simulink model "Mass_Springs_Systems"  (R2021b)
settings: Solver=ode4  StartTime=0.0  StopTime=20  FixedStep=.001  RelTol=1e-3  AbsTol=1e-3  EnableMultiTasking=on
model workspace (MAT data in the model file):
  cslide = 0.25
  iz = [0.192  0.091; 0.207  0.094; 0.221  0.104; 0.238  0.118; 0.251  0.141; 0.262  0.168; 0.268  0.205; 0.27  0.242; 0.267  0.277; 0.262  0.308; 0.246  0.348; 0.232  0.369; 0.206  0.39; 0.185  0.39; 0.16  0.377; 0.137  0.349; 0.126  0.325; 0.118  0.297; 0.114  0.265; 0.113  0.237; 0.118  0.191; 0.128  0.156; 0.139  0.13; 0.156  0.107; 0.175  0.096]
  m1 = 0
  m2 = 0
  m3 = 0
  one = [0.064  0.072; 0.088  0.03; 0.169  0.03; 0.168  0.458; 0.129  0.458; 0.128  0.073]
  smiData.RigidTransform.translation = [-21.5561986301 -14.8674859839 15.0728144895]
  smiData.RigidTransform.angle = 0
  smiData.RigidTransform.axis = [0 0 0]
  smiData.RigidTransform.ID = 'RootGround[rack-1]'
  smiData.Solid.mass = 0.0200061588425
  smiData.Solid.CoM = [0 0.838779102261 -0.00603396973069]
  smiData.Solid.MoI = [0.670200057653 0.669872690066 0.00366172739385]
  smiData.Solid.PoI = [5.56695055283e-05 0 0]
  smiData.Solid.color = [0.792156862745 0.819607843137 0.933333333333]
  smiData.Solid.opacity = 1
  smiData.Solid.ID = 'rack*:*Default'
  three = [0.252  0.12; 0.239  0.091; 0.214  0.068; 0.179  0.053; 0.14  0.052; 0.107  0.064; 0.083  0.082; 0.065  0.121; 0.075  0.155; 0.102  0.176; 0.129  0.188; 0.163  0.194; 0.182  0.194; 0.183  0.24; 0.131  0.247; 0.099  0.256; 0.068  0.28; 0.048  0.313; 0.047  0.345; 0.055  0.378; 0.084  0.41; 0.127  0.429; 0.179  0.43; 0.214  0.419; 0.246  0.396; 0.26  0.368; 0.269  0.344; 0.311  0.344; 0.303  0.374; 0.29  0.409; 0.262  0.442; 0.23  0.463; 0.18  0.475; 0.137  0.476; 0.097  0.465; 0.057  0.441; 0.028  0.411; 0.011  0.374; 0.006  0.353; 0.01  0.295; 0.028  0.258; 0.05  0.233; 0.08  0.214; 0.06  0.196; 0.041  0.175; 0.029  0.135; 0.029  0.104; 0.043  0.066; 0.074  0.032; 0.106  0.015; 0.147  0.006; 0.187  0.007; 0.223  0.021; 0.255  0.044; 0.278  0.081; 0.294  0.119]
  two = [0.081  0.154; 0.042  0.154; 0.05  0.108; 0.06  0.085; 0.082  0.055; 0.106  0.033; 0.135  0.02; 0.161  0.013; 0.194  0.014; 0.226  0.02; 0.253  0.032; 0.279  0.054; 0.297  0.083; 0.305  0.109; 0.309  0.141; 0.306  0.168; 0.299  0.189; 0.281  0.221; 0.242  0.271; 0.119  0.401; 0.315  0.403; 0.314  0.445; 0.027  0.446; 0.242  0.214; 0.263  0.177; 0.272  0.145; 0.264  0.106; 0.243  0.079; 0.208  0.059; 0.185  0.058; 0.162  0.06; 0.133  0.067; 0.12  0.076; 0.102  0.092; 0.088  0.119; 0.085  0.134]
  xy_simple = [39.1661  19.7032018238; 3.8339  19.7032; -0.28263658  19.7032; -0.28263658  0; 43  0; 43  19.7032]
  zero = [0.2  0.026; 0.245  0.033; 0.288  0.063; 0.316  0.099; 0.335  0.149; 0.345  0.197; 0.347  0.246; 0.344  0.292; 0.338  0.339; 0.324  0.384; 0.3  0.429; 0.269  0.456; 0.223  0.475; 0.173  0.475; 0.132  0.46; 0.097  0.426; 0.072  0.383; 0.062  0.338; 0.058  0.289; 0.058  0.242; 0.059  0.192; 0.068  0.145; 0.083  0.102; 0.111  0.062; 0.149  0.037]
undefined symbols (not defined in the file): _Default_sldprt, A, b3ih, d1, d2, ha, sigbuilder_block, Unbalanced_CartV1, X, Y, Z
libraries: sm_lib x7356, nesl_utility x64, simulink x2
(part 1 of 150)
settings Model: Creator=HP Owner  LastModifiedBy=atekes
settings SolverCC: AutoScaleAbsTol=off  AlgebraicLoopSolver=TrustRegion
settings DataIOCC: MaxDataPoints=10000
settings OptimizationCC: LifeSpan=inf
settings DebuggingCC: AllowSymbolicDim=off  SFUnexpectedBacktrackingDiag=warning  SFNoUnconditionalDefaultTransitionDiag=warning  SFExecutionAtInitializationDiag=none  SFMachineParentedDataDiag=warning  ArithmeticOperatorsInVariantConditions=warning
settings SFSimCC: SimUseLocalCustomCode=off  CustomCodeUndefinedFunction=UseInterfaceOnly
settings RTWCC: RTWUseLocalCustomCode=off
settings CodeAppCC: StateflowObjectComments=on
settings GRTTargetCC: TargetLangStandard=C89/C90 (ANSI)
settings ConfigComp: CovMetricSettings=dw  CovSaveCumulativeToWorkspaceVar=on  CovSaveSingleToWorkspaceVar=on  CovExternalEMLEnable=off  CovSFcnEnable=off
settings SimscapeCC: SimscapeLogType=all  SimscapeLogSimulationStatistics=on  SimscapeLogDataHistory=10000

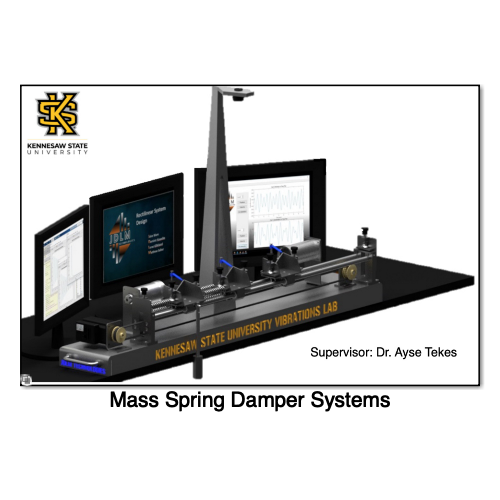
[thumbnail: Simulink's stored preview of the top-level diagram]
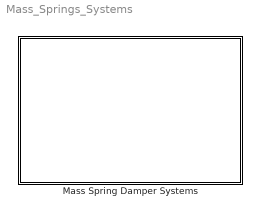
== system Mass_Springs_Systems ==
  Mass Spring Damper Systems : Subsystem  Variant=on  VariantControlMode=label  VariantControl=MS  LabelModeActiveChoice=TRU
      mask Display: image('$imagefile'); % Use "Edit Image" on toolstrip to change.
